simulink model "Lab_4_Simulink"  (R2025a)
settings: Solver=VariableStepAuto  StartTime=0.0  StopTime=0.1  MaxStep=1e-5  RelTol=1e-3
undefined symbols (not defined in the file): alpha
libraries: spsDiodeLib x12, spsDetailedThyristorLib x9, spsACVoltageSourceLib x8, spsMeanLib x6, spsSeriesRLCBranchLib x6, spsVoltageMeasurementLib x6, sps_lib x5, spsGroundLib x1
settings Model: Creator=MRINAL  LastModifiedBy=MRINAL

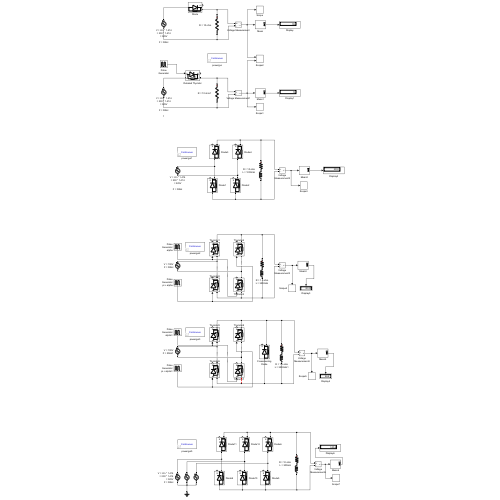
[thumbnail: Simulink's stored preview of the top-level diagram]
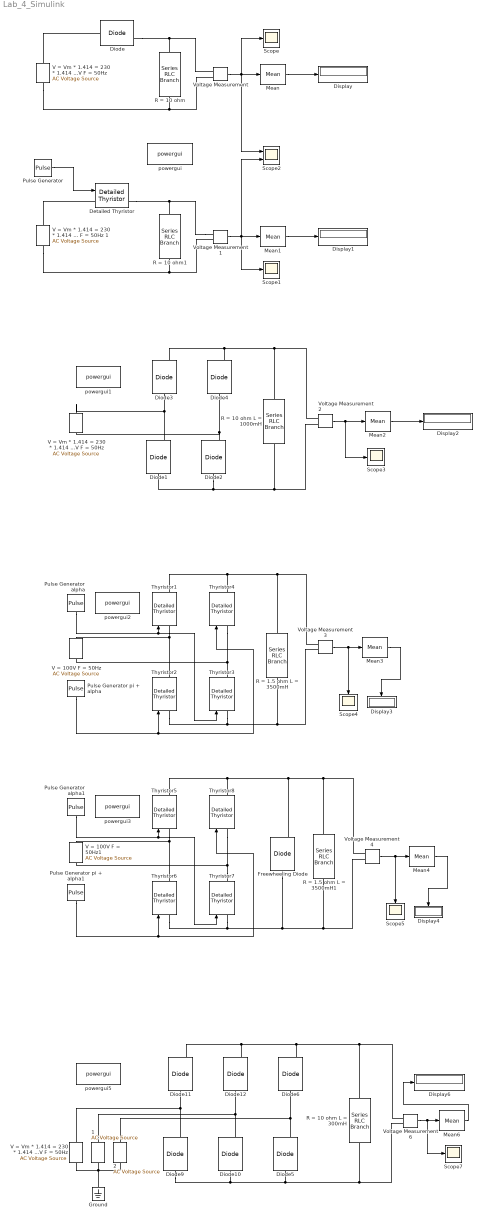
== system Lab_4_Simulink ==
  1 : spsACVoltageSourceLib/AC Voltage Source  Amplitude=325  Phase=0  Frequency=50  SampleTime=0  Measurements=None  BusType=swing  Pref=10e3  Qref=0  Qmin=-inf  Qmax=+inf
  2 : spsACVoltageSourceLib/AC Voltage Source  Amplitude=325  Phase=120  Frequency=50  SampleTime=0  Measurements=None  BusType=swing  Pref=10e3  Qref=0  Qmin=-inf  Qmax=+inf
  Detailed Thyristor : spsDetailedThyristorLib/Detailed Thyristor  Ron=0.001  Lon=1e-3  Vf=0.8  IL=0.1  Tq=100e-6  IC=0  Rs=500  Cs=250e-9  Measurements=on
      settings: LibrarySourceBlock=sps_lib/Power Electronics/Detailed Thyristor
  Diode{,1..6,9..12} (11 alike) : spsDiodeLib/Diode  Ron=0.001  Lon=0  Vf=0.8  IC=0  UseSnubber=0  Rs=500  Cs=250e-9  Measurements=on
  Display{,1..4,6} (6 alike) : Display
  Freewheeling Diode : spsDiodeLib/Diode  Ron=0.001  Lon=0  Vf=0.8  IC=0  UseSnubber=0  Rs=500  Cs=250e-9  Measurements=on
  Ground : spsGroundLib/Ground  LConnTagsString=a
  Mean{,1..4,6} (6 alike) : spsMeanLib/Mean  Freq=50  Vinit=0  Ts=0
  Pulse Generator : DiscretePulseGenerator  PulseType=Time based  Period=0.02  PulseWidth=5  PhaseDelay=alpha/350 * 0.02
  Pulse Generator alpha : DiscretePulseGenerator  PulseType=Time based  Period=0.02  PulseWidth=5  PhaseDelay=(alpha)/360 * 0.02
  Pulse Generator alpha1 : DiscretePulseGenerator  PulseType=Time based  Period=0.02  PulseWidth=5  PhaseDelay=(alpha)/360 * 0.02
  Pulse Generator pi + alpha : DiscretePulseGenerator  PulseType=Time based  Period=0.02  PulseWidth=5  PhaseDelay=(180 + alpha)/360 * 0.02
  Pulse Generator pi + alpha1 : DiscretePulseGenerator  PulseType=Time based  Period=0.02  PulseWidth=5  PhaseDelay=(180 + alpha)/360 * 0.02
  R = 1.5 ohm L = 3500mH : spsSeriesRLCBranchLib/Series RLC Branch  LConnTagsString=__new0  RConnTagsString=__new0  BranchType=RL  Resistance=1.5  Inductance=3500e-3  SetiL0=off  InitialCurrent=0  Capacitance=1e-6  Setx0=off  InitialVoltage=0  Measurements=None
  R = 1.5 ohm L = 3500mH1 : spsSeriesRLCBranchLib/Series RLC Branch  LConnTagsString=__new0  RConnTagsString=__new0  BranchType=RL  Resistance=1.5  Inductance=3500e-3  SetiL0=off  InitialCurrent=0  Capacitance=1e-6  Setx0=off  InitialVoltage=0  Measurements=None
  R = 10 ohm : spsSeriesRLCBranchLib/Series RLC Branch  LConnTagsString=__new0  RConnTagsString=__new0  BranchType=R  Resistance=10  Inductance=1e-3  SetiL0=off  InitialCurrent=0  Capacitance=1e-6  Setx0=off  InitialVoltage=0  Measurements=None
  R = 10 ohm L = 1000mH : spsSeriesRLCBranchLib/Series RLC Branch  LConnTagsString=__new0  RConnTagsString=__new0  BranchType=RL  Resistance=10  Inductance=1000e-3  SetiL0=off  InitialCurrent=0  Capacitance=1e-6  Setx0=off  InitialVoltage=0  Measurements=None
  R = 10 ohm L = 300mH : spsSeriesRLCBranchLib/Series RLC Branch  LConnTagsString=__new0  RConnTagsString=__new0  BranchType=RL  Resistance=10  Inductance=300e-3  SetiL0=off  InitialCurrent=0  Capacitance=1e-6  Setx0=off  InitialVoltage=0  Measurements=None
  R = 10 ohm1 : spsSeriesRLCBranchLib/Series RLC Branch  LConnTagsString=__new0  RConnTagsString=__new0  BranchType=R  Resistance=10  Inductance=1e-3  SetiL0=off  InitialCurrent=0  Capacitance=1e-6  Setx0=off  InitialVoltage=0  Measurements=None
  Scope{,1,3..5,7} (6 alike) : Scope
      Scope settings: Title=230929228_Mrinal_Kumar  ActiveDisplayYMinimum=-1  ActiveDisplayYMaximum=1  YLabel=Voltage
      Scope1 settings: Title=230929228_Mrinal_Kumar  ActiveDisplayYMinimum=-40.802375808005635  ActiveDisplayYMaximum=364.71968919659759  YLabel=Voltage
      Scope3 settings: Title=230929228_Mrinal_Kumar  ActiveDisplayYMinimum=-42.238384502276247  ActiveDisplayYMaximum=364.0239143778179  YLabel=Voltage  DataLoggingVariableName=ScopeData3
      Scope4 settings: Title=230929228_Mrinal_Kumar  ActiveDisplayYMinimum=-1  ActiveDisplayYMaximum=1  YLabel=Voltage  DataLoggingVariableName=ScopeData4
      Scope5 settings: Title=230929228_Mrinal_Kumar  ActiveDisplayYMinimum=-13.201436024344128  ActiveDisplayYMaximum=110.80005885802862  YLabel=Voltage  DataLoggingVariableName=ScopeData5
      Scope7 settings: Title=230929228_Mrinal_Kumar  ActiveDisplayYMinimum=0  ActiveDisplayYMaximum=570.7495  YLabel=Voltage  DataLoggingVariableName=ScopeData7
  Scope2 : Scope  NumInputPorts=2
      settings: Title=230929228_Mrinal_Kumar  ActiveDisplayYMinimum=-40.802389110380105  ActiveDisplayYMaximum=364.7198023540692  YLabel=Voltage  DataLoggingVariableName=ScopeData2
  Thyristor{1..8} (8 alike) : spsDetailedThyristorLib/Detailed Thyristor  Ron=0.001  Lon=1e-3  Vf=0.8  IL=0.1  Tq=100e-6  IC=0  Rs=500  Cs=250e-9  Measurements=on
      settings: LibrarySourceBlock=sps_lib/Power Electronics/Detailed Thyristor
  V = 100V F = 50Hz : spsACVoltageSourceLib/AC Voltage Source  Amplitude=100  Phase=0  Frequency=50  SampleTime=0  Measurements=None  BusType=swing  Pref=10e3  Qref=0  Qmin=-inf  Qmax=+inf
  V = 100V F = 50Hz1 : spsACVoltageSourceLib/AC Voltage Source  Amplitude=100  Phase=0  Frequency=50  SampleTime=0  Measurements=None  BusType=swing  Pref=10e3  Qref=0  Qmin=-inf  Qmax=+inf
  V = Vm * 1.414 = 230 * 1.414 = 325V F = 50Hz : spsACVoltageSourceLib/AC Voltage Source  Amplitude=325  Phase=0  Frequency=50  SampleTime=0  Measurements=None  BusType=swing  Pref=10e3  Qref=0  Qmin=-inf  Qmax=+inf
  "V = Vm * 1.414 = 230 * 1.414 = 325V F = 50Hz " : spsACVoltageSourceLib/AC Voltage Source  Amplitude=325  Phase=0  Frequency=50  SampleTime=0  Measurements=None  BusType=swing  Pref=10e3  Qref=0  Qmin=-inf  Qmax=+inf
  V = Vm * 1.414 = 230 * 1.414 = 325V F = 50Hz 1 : spsACVoltageSourceLib/AC Voltage Source  Amplitude=325  Phase=0  Frequency=50  SampleTime=0  Measurements=None  BusType=swing  Pref=10e3  Qref=0  Qmin=-inf  Qmax=+inf
  V = Vm * 1.414 = 230 * 1.414 = 325V F = 50Hz : spsACVoltageSourceLib/AC Voltage Source  Amplitude=325  Phase=-120  Frequency=50  SampleTime=0  Measurements=None  BusType=swing  Pref=10e3  Qref=0  Qmin=-inf  Qmax=+inf
  Voltage Measurement{,1..4,6} (6 alike) : spsVoltageMeasurementLib/Voltage Measurement  PhasorSimulation=off  OutputType=Complex  PSBequivalent=0
  powergui{,1..3,5} (5 alike) : sps_lib/powergui  Priority=1  SimulationMode=Continuous  SampleTime=50e-6  frequency=60  Iterations=50  frequencyindice=50  Pbase=100e6  ErrMax=1e-4  UnitsV=kV  UnitsW=MW  buscounter=0  FunctionMessages=off  echomessages=off  EnableUseOfTLC=off  CurrentSourceSwitches=off  DisableSnubberDevices=off  DisableRonSwitches=off  DisableVfSwitches=off  DisplayEquations=off  AutomaticDiscreteSolvers=off  SolverType=Tustin/Backward Euler (TBE)  Interpol=off  ExternalGateDelay=off  methode=off  Ts=100  x0status=zero  SPID=on  SwTol=0  HookPort=off  NonlinearTolerance=1e-4  nMaxIteration=100  ContinueOnMaxIteration=off  RestoreLinks=warning  ResistiveCurrentMeasurement=off  Frange=[0:2:500]  Ylog=off  Xlog=on  ShowGrid=off  save=off  variable=ZData  structure=0  ZoomFFT=off  StartTime=0.0  cycles=1  DisplayStyle=1  fundamental=60  FreqAxis=off  MaxFrequency=1000  frequencyindicesteady=1  RmsSteady=1  display=off
  wires:
  Voltage Measurement/1 -> Mean/1, Scope2/1, Scope/1
  Mean/1 -> Display/1
  Mean1/1 -> Display1/1
  Voltage Measurement1/1 -> Scope1/1, Mean1/1, Scope2/2
  Pulse Generator/1 -> Detailed Thyristor/1
  Voltage Measurement2/1 -> Scope3/1, Mean2/1
  Mean2/1 -> Display2/1
  Voltage Measurement3/1 -> Scope4/1, Mean3/1
  Mean3/1 -> Display3/1
  Pulse Generator alpha/1 -> Thyristor1/1, Thyristor3/1
  Pulse Generator pi + alpha/1 -> Thyristor2/1, Thyristor4/1
  Pulse Generator alpha1/1 -> Thyristor5/1, Thyristor7/1
  Pulse Generator pi + alpha1/1 -> Thyristor6/1, Thyristor8/1
  Mean4/1 -> Display4/1
  Voltage Measurement4/1 -> Scope5/1, Mean4/1
  Mean6/1 -> Display6/1
  Voltage Measurement6/1 -> Mean6/1, Scope7/1
  connections:
  R = 10 ohm/LConn1 -- Diode/RConn1 -- Voltage Measurement/LConn1
  Voltage Measurement/LConn2 -- "V = Vm * 1.414 = 230 * 1.414 = 325V F = 50Hz "/LConn1 -- R = 10 ohm/RConn1
  "V = Vm * 1.414 = 230 * 1.414 = 325V F = 50Hz "/RConn1 -- Diode/LConn1
  Voltage Measurement1/LConn1 -- Detailed Thyristor/RConn1 -- R = 10 ohm1/LConn1
  Voltage Measurement1/LConn2 -- V = Vm * 1.414 = 230 * 1.414 = 325V F = 50Hz 1/LConn1 -- R = 10 ohm1/RConn1
  V = Vm * 1.414 = 230 * 1.414 = 325V F = 50Hz 1/RConn1 -- Detailed Thyristor/LConn1
  Diode2/RConn1 -- V = Vm * 1.414 = 230 * 1.414 = 325V F = 50Hz/LConn1 -- Diode4/LConn1
  Diode1/RConn1 -- V = Vm * 1.414 = 230 * 1.414 = 325V F = 50Hz/RConn1 -- Diode3/LConn1
  R = 10 ohm L = 1000mH/LConn1 -- Voltage Measurement2/LConn1 -- Diode3/RConn1 -- Diode4/RConn1
  Diode2/LConn1 -- Diode1/LConn1 -- R = 10 ohm L = 1000mH/RConn1 -- Voltage Measurement2/LConn2
  Voltage Measurement3/LConn2 -- Thyristor3/LConn1 -- Thyristor2/LConn1 -- R = 1.5 ohm L = 3500mH/RConn1
  Voltage Measurement3/LConn1 -- Thyristor4/RConn1 -- Thyristor1/RConn1 -- R = 1.5 ohm L = 3500mH/LConn1
  Thyristor1/LConn1 -- Thyristor2/RConn1 -- V = 100V F = 50Hz/RConn1
  Thyristor4/LConn1 -- V = 100V F = 50Hz/LConn1 -- Thyristor3/RConn1
  Thyristor8/RConn1 -- Freewheeling Diode/RConn1 -- R = 1.5 ohm L = 3500mH1/LConn1 -- Voltage Measurement4/LConn1 -- Thyristor5/RConn1
  Thyristor7/RConn1 -- V = 100V F = 50Hz1/LConn1 -- Thyristor8/LConn1
  Thyristor5/LConn1 -- Thyristor6/RConn1 -- V = 100V F = 50Hz1/RConn1
  R = 1.5 ohm L = 3500mH1/RConn1 -- Thyristor7/LConn1 -- Thyristor6/LConn1 -- Freewheeling Diode/LConn1 -- Voltage Measurement4/LConn2
  Diode10/RConn1 -- 1/RConn1 -- Diode12/LConn1
  Diode9/RConn1 -- V = Vm * 1.414 = 230 * 1.414 = 325V F = 50Hz/RConn1 -- Diode11/LConn1
  Voltage Measurement6/LConn1 -- Diode11/RConn1 -- Diode12/RConn1 -- Diode6/RConn1 -- R = 10 ohm L = 300mH/LConn1
  Voltage Measurement6/LConn2 -- Diode5/LConn1 -- Diode10/LConn1 -- Diode9/LConn1 -- R = 10 ohm L = 300mH/RConn1
  Diode5/RConn1 -- 2/RConn1 -- Diode6/LConn1
  Ground/LConn1 -- 1/LConn1 -- V = Vm * 1.414 = 230 * 1.414 = 325V F = 50Hz/LConn1 -- 2/LConn1
